simulink model "lsb"  (R2024b)
settings: Solver=FixedStepAuto  StartTime=0.0  StopTime=8  FixedStep=1/100  RelTol=1e-3
settings Model: Creator=sucho  LastModifiedBy=sucho
settings RTWCC: GPUComputeCapability=3.5

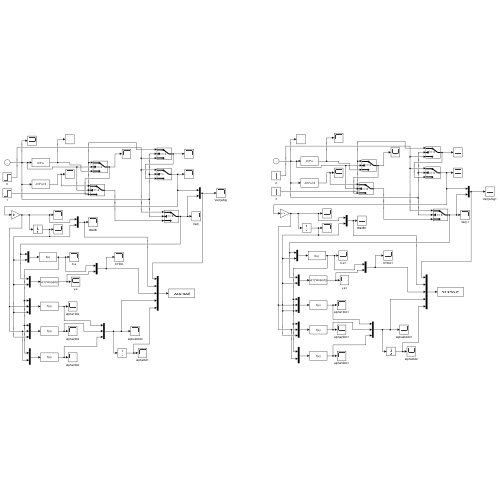
[thumbnail: Simulink's stored preview of the top-level diagram]
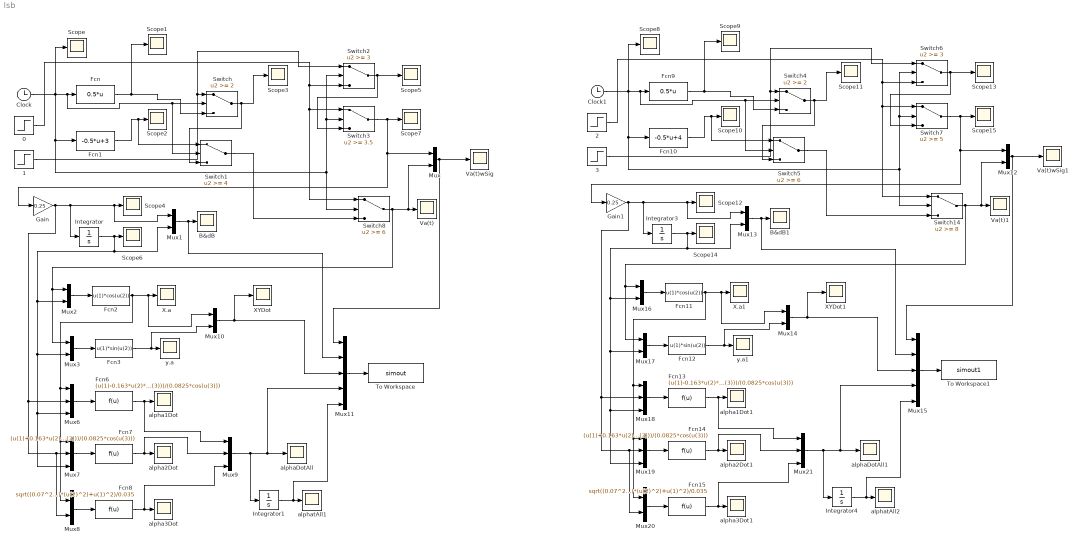
== system lsb ==
  0 : Step  Time=0  After=0  SampleTime=0
  1 : Step  Time=0  SampleTime=0
  2 : Step  Time=0  After=0  SampleTime=0
  3 : Step  Time=0  SampleTime=0
  B&dB : Scope
  B&dB1 : Scope
  Clock : Clock
  Clock1 : Clock
  Fcn : Fcn  Expr=0.5*u
  Fcn1 : Fcn  Expr=-0.5*u+3
  Fcn10 : Fcn  Expr=-0.5*u+4
  Fcn11 : Fcn  Expr=u(1)*cos(u(2))
  Fcn12 : Fcn  Expr=u(1)*sin(u(2))
  Fcn13 : Fcn  Expr=(u(1)-0.163*u(2)*cos(u(3)))/(0.0825*cos(u(3)))
  Fcn14 : Fcn  Expr=(u(1)+0.163*u(2)*cos(u(3)))/(0.0825*cos(u(3)))
  Fcn15 : Fcn  Expr=sqrt((0.07^2)*(u(2)^2)+u(1)^2)/0.035
  Fcn2 : Fcn  Expr=u(1)*cos(u(2))
  Fcn3 : Fcn  Expr=u(1)*sin(u(2))
  Fcn6 : Fcn  Expr=(u(1)-0.163*u(2)*cos(u(3)))/(0.0825*cos(u(3)))
  Fcn7 : Fcn  Expr=(u(1)+0.163*u(2)*cos(u(3)))/(0.0825*cos(u(3)))
  Fcn8 : Fcn  Expr=sqrt((0.07^2)*(u(2)^2)+u(1)^2)/0.035
  Fcn9 : Fcn  Expr=0.5*u
  Gain : Gain  Gain=0.25
  Gain1 : Gain  Gain=0.25
  Integrator{,1,3..4} (4 alike) : Integrator
  Mux{,1..3,8,10,12..14,16..17,20} (12 alike) : Mux  Inputs=2
  Mux11 : Mux  Inputs=5
  Mux15 : Mux  Inputs=5
  Mux{6..7,9,18..19,21} (6 alike) : Mux  Inputs=3
  Scope{,1..15} (16 alike) : Scope
  Switch : Switch  Threshold=2  SaturateOnIntegerOverflow=off  InputSameDT=off
  Switch1 : Switch  Threshold=4  SaturateOnIntegerOverflow=off  InputSameDT=off
  Switch14 : Switch  Threshold=8  SaturateOnIntegerOverflow=off  InputSameDT=off
  Switch2 : Switch  Threshold=3  SaturateOnIntegerOverflow=off  InputSameDT=off
  Switch3 : Switch  Threshold=3.5  SaturateOnIntegerOverflow=off  InputSameDT=off
  Switch4 : Switch  Threshold=2  SaturateOnIntegerOverflow=off  InputSameDT=off
  Switch5 : Switch  Threshold=6  SaturateOnIntegerOverflow=off  InputSameDT=off
  Switch6 : Switch  Threshold=3  SaturateOnIntegerOverflow=off  InputSameDT=off
  Switch7 : Switch  Threshold=5  SaturateOnIntegerOverflow=off  InputSameDT=off
  Switch8 : Switch  Threshold=6  SaturateOnIntegerOverflow=off  InputSameDT=off
  To Workspace : ToWorkspace  VariableName=simout  SaveFormat=Timeseries  SampleTime=-1
  To Workspace1 : ToWorkspace  VariableName=simout1  SaveFormat=Timeseries  SampleTime=-1
  Va(t) : Scope
  Va(t)1 : Scope
  Va(t)wSig : Scope
  Va(t)wSig1 : Scope
  X.a : Scope
  X.a1 : Scope
  XYDot : Scope
  XYDot1 : Scope
  alpha1Dot : Scope
  alpha1Dot1 : Scope
  alpha2Dot : Scope
  alpha2Dot1 : Scope
  alpha3Dot : Scope
  alpha3Dot1 : Scope
  alphaDotAll : Scope
  alphaDotAll1 : Scope
  alphatAll1 : Scope
  alphatAll2 : Scope
  y.a : Scope
  y.a1 : Scope
  wires:
  Fcn/1 -> Switch/3, Scope1/1
  Clock/1 -> Scope/1, Fcn1/1, Switch8/2, Switch3/2, Switch2/2, Switch1/2, Switch/2, Fcn/1
  Fcn1/1 -> Switch1/1, Scope2/1
  1/1 -> Switch2/1, Switch/1
  Switch/1 -> Switch1/3, Scope3/1
  Switch1/1 -> Switch8/3
  0/1 -> Switch3/1, Switch8/1, Switch2/3
  Switch2/1 -> Switch3/3, Scope5/1
  Switch3/1 -> Gain/1, Mux/1, Scope7/1
  Mux/1 -> Mux11/1, Va(t)wSig/1
  Gain/1 -> Integrator/1, Mux1/1, Scope4/1, Mux6/2, Mux7/2, Mux8/2
  Integrator/1 -> Mux2/2, Mux7/3, Mux6/3, Mux3/2, Mux1/2, Scope6/1
  Mux1/1 -> Mux11/2, B&dB/1
  Switch8/1 -> Mux2/1, Mux3/1, Mux/2, Va(t)/1
  Mux2/1 -> Fcn2/1
  Fcn2/1 -> Mux8/1, Mux7/1, Mux6/1, Mux10/1, X.a/1
  Mux3/1 -> Fcn3/1
  Fcn3/1 -> Mux10/2, y.a/1
  Mux6/1 -> Fcn6/1
  Fcn6/1 -> Mux9/1, alpha1Dot/1
  Mux7/1 -> Fcn7/1
  Fcn7/1 -> Mux9/2, alpha2Dot/1
  Mux8/1 -> Fcn8/1
  Fcn8/1 -> Mux9/3, alpha3Dot/1
  Mux9/1 -> Integrator1/1, alphaDotAll/1, Mux11/4
  Integrator1/1 -> Mux11/5, alphatAll1/1
  Mux10/1 -> Mux11/3, XYDot/1
  Mux11/1 -> To Workspace/1
  Mux14/1 -> Mux15/3, XYDot1/1
  Mux15/1 -> To Workspace1/1
  Integrator4/1 -> Mux15/5, alphatAll2/1
  Mux21/1 -> Integrator4/1, alphaDotAll1/1, Mux15/4
  Mux20/1 -> Fcn15/1
  Fcn11/1 -> Mux20/1, Mux19/1, Mux18/1, Mux14/1, X.a1/1
  Fcn10/1 -> Switch5/1, Scope10/1
  Mux19/1 -> Fcn14/1
  Fcn12/1 -> Mux14/2, y.a1/1
  Fcn14/1 -> Mux21/2, alpha2Dot1/1
  Switch6/1 -> Switch7/3, Scope13/1
  Integrator3/1 -> Mux16/2, Mux19/3, Mux18/3, Mux17/2, Mux13/2, Scope14/1
  Mux16/1 -> Fcn11/1
  Mux18/1 -> Fcn13/1
  Fcn9/1 -> Switch4/3, Scope9/1
  Mux13/1 -> Mux15/2, B&dB1/1
  Mux17/1 -> Fcn12/1
  3/1 -> Switch6/1, Switch4/1
  2/1 -> Switch7/1, Switch14/1, Switch6/3
  Clock1/1 -> Scope8/1, Fcn10/1, Switch14/2, Switch7/2, Switch6/2, Switch5/2, Switch4/2, Fcn9/1
  Switch7/1 -> Gain1/1, Mux12/1, Scope15/1
  Fcn13/1 -> Mux21/1, alpha1Dot1/1
  Mux12/1 -> Mux15/1, Va(t)wSig1/1
  Switch4/1 -> Switch5/3, Scope11/1
  Gain1/1 -> Integrator3/1, Mux13/1, Scope12/1, Mux18/2, Mux19/2, Mux20/2
  Switch5/1 -> Switch14/3
  Switch14/1 -> Mux16/1, Mux17/1, Mux12/2, Va(t)1/1
  Fcn15/1 -> Mux21/3, alpha3Dot1/1
